simulink model "pand"  (R2023b)
settings: Solver=VariableStepAuto  StartTime=0.0  StopTime=10  RelTol=1e-3
libraries: simulink x1
settings Model: Creator=asus  LastModifiedBy=asus

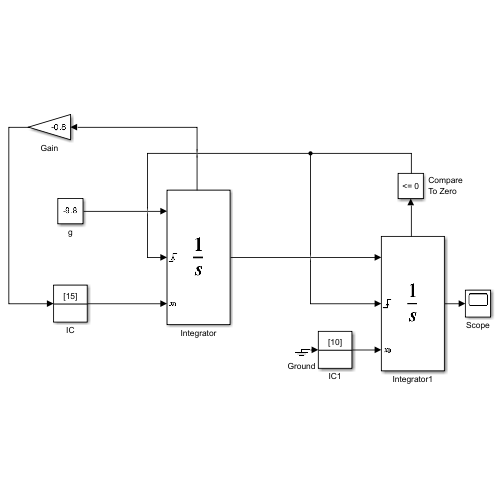
[thumbnail: Simulink's stored preview of the top-level diagram]
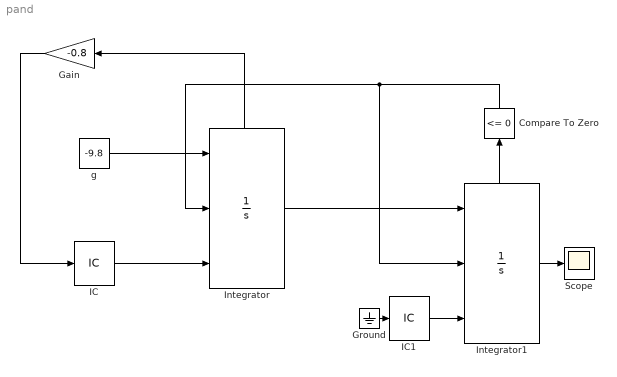
== system pand ==
  Compare To Zero : simulink/Logic and Bit Operations/Compare To Zero  relop=<=  OutDataTypeStr=boolean
  Gain : Gain  Gain=-0.8
  Ground : Ground
  IC : InitialCondition  Value=15
  IC1 : InitialCondition  Value=10
  Integrator : Integrator  ExternalReset=rising  InitialConditionSource=external  ShowStatePort=on
  Integrator1 : Integrator  ExternalReset=rising  InitialConditionSource=external  ShowStatePort=on
  Scope : Scope
  g : Constant  Value=-9.8
  wires:
  g/1 -> Integrator/1
  IC/1 -> Integrator/3
  Integrator/1 -> Integrator1/1
  Integrator1/State -> Compare To Zero/1
  Compare To Zero/1 -> Integrator1/2, Integrator/2
  Gain/1 -> IC/1
  IC1/1 -> Integrator1/3
  Ground/1 -> IC1/1
  Integrator1/1 -> Scope/1
  Integrator/State -> Gain/1
